simulink model "sim_2"  (R2013b)
settings: Solver=ode3  StartTime=0.0  StopTime=2  MaxStep=0.01  RelTol=1e-3
settings Model: Creator=Ali  LastModifiedBy=Ali

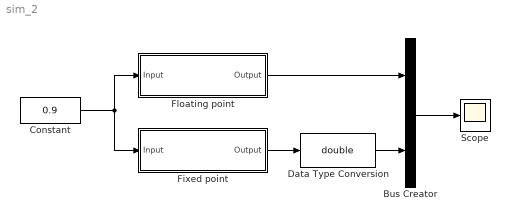
== system sim_2 ==
  Bus Creator : BusCreator  Inputs=2
  Constant : Constant  Value=0.9  SampleTime=Inf
  Data Type Conversion : DataTypeConversion  OutDataTypeStr=double
  Fixed point : Subsystem  Tag=FilterWizardSubSystem
      settings: ErrorFcn=dspFilterRealizedInBasicElemsAlgLoopErrFcnCallback
  Floating point : Subsystem  Tag=FilterWizardSubSystem
      settings: ErrorFcn=dspFilterRealizedInBasicElemsAlgLoopErrFcnCallback
  Scope : Scope
  wires:
  Constant/1 -> Floating point/1(Input), Fixed point/1(Input)
  Floating point/1(Output) -> Bus Creator/1
  Fixed point/1(Output) -> Data Type Conversion/1
  Bus Creator/1 -> Scope/1
  Data Type Conversion/1 -> Bus Creator/2

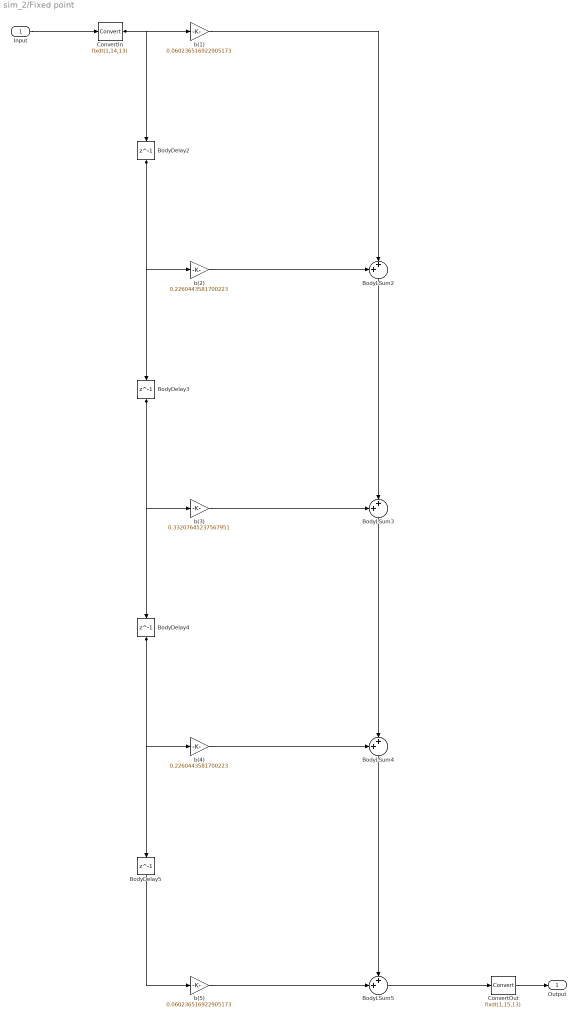
== system sim_2/Fixed point ==
  Input : Inport
  BodyDelay{2..5} (4 alike) : Delay  DelayLength=1  InitialCondition=0  InputProcessing=Columns as channels (frame based)
  BodyLSum{2..5} (4 alike) : Sum  Inputs=++|  AccumDataTypeStr=fixdt(1,22,21)  OutDataTypeStr=fixdt(1,22,21)  RndMeth=Convergent
  ConvertIn : DataTypeConversion  OutDataTypeStr=fixdt(1,14,13)  RndMeth=Nearest  SaturateOnIntegerOverflow=on
  ConvertOut : DataTypeConversion  OutDataTypeStr=fixdt(1,15,13)  RndMeth=Convergent
  b(1) : Gain  Gain=0.060236516922905173  ParamDataTypeStr=fixdt(1,9,8)  OutDataTypeStr=fixdt(1,21,21)  RndMeth=Convergent
  b(2) : Gain  Gain=0.2260443581700223  ParamDataTypeStr=fixdt(1,9,8)  OutDataTypeStr=fixdt(1,21,21)  RndMeth=Convergent
  b(3) : Gain  Gain=0.33207645237567951  ParamDataTypeStr=fixdt(1,9,8)  OutDataTypeStr=fixdt(1,21,21)  RndMeth=Convergent
  b(4) : Gain  Gain=0.2260443581700223  ParamDataTypeStr=fixdt(1,9,8)  OutDataTypeStr=fixdt(1,21,21)  RndMeth=Convergent
  b(5) : Gain  Gain=0.060236516922905173  ParamDataTypeStr=fixdt(1,9,8)  OutDataTypeStr=fixdt(1,21,21)  RndMeth=Convergent
  Output : Outport
  wires:
  Input/1 -> ConvertIn/1
  b(1)/1 -> BodyLSum2/2
  ConvertIn/1 -> b(1)/1, BodyDelay2/1
  BodyDelay2/1 -> b(2)/1, BodyDelay3/1
  b(2)/1 -> BodyLSum2/1
  BodyLSum2/1 -> BodyLSum3/2
  BodyDelay3/1 -> b(3)/1, BodyDelay4/1
  b(3)/1 -> BodyLSum3/1
  BodyLSum3/1 -> BodyLSum4/2
  BodyDelay4/1 -> b(4)/1, BodyDelay5/1
  b(4)/1 -> BodyLSum4/1
  BodyLSum4/1 -> BodyLSum5/1
  BodyDelay5/1 -> b(5)/1
  b(5)/1 -> BodyLSum5/2
  BodyLSum5/1 -> ConvertOut/1
  ConvertOut/1 -> Output/1

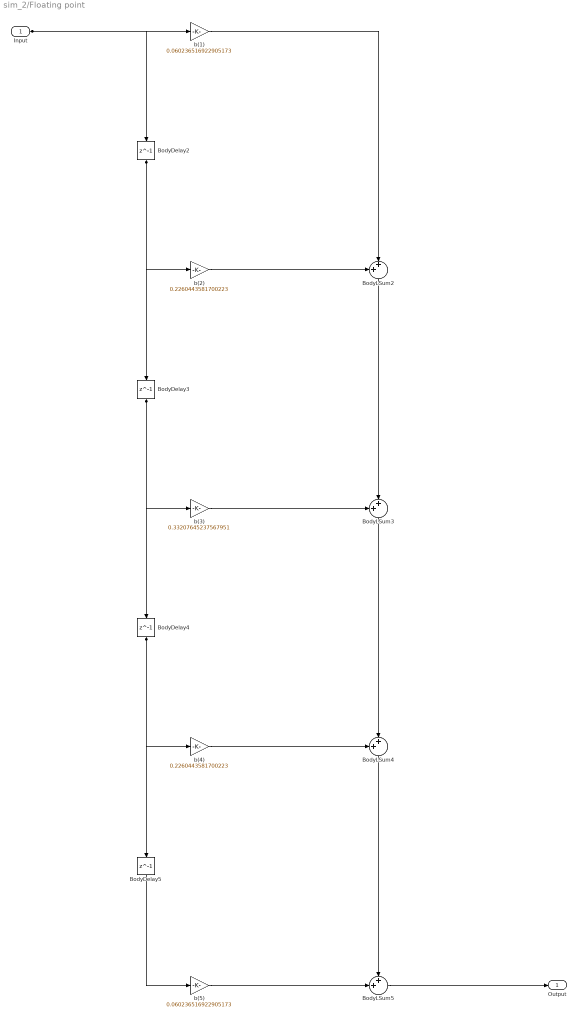
== system sim_2/Floating point ==
  Input : Inport
  BodyDelay{2..5} (4 alike) : Delay  DelayLength=1  InitialCondition=0  InputProcessing=Columns as channels (frame based)
  BodyLSum{2..5} (4 alike) : Sum  Inputs=++|  RndMeth=Nearest  SaturateOnIntegerOverflow=on  OutDataTypeStr=Inherit: Same as first input
  b(1) : Gain  Gain=0.060236516922905173  ParamDataTypeStr=double  RndMeth=Nearest  SaturateOnIntegerOverflow=on  OutDataTypeStr=Inherit: Same as input
  b(2) : Gain  Gain=0.2260443581700223  ParamDataTypeStr=double  RndMeth=Nearest  SaturateOnIntegerOverflow=on  OutDataTypeStr=Inherit: Same as input
  b(3) : Gain  Gain=0.33207645237567951  ParamDataTypeStr=double  RndMeth=Nearest  SaturateOnIntegerOverflow=on  OutDataTypeStr=Inherit: Same as input
  b(4) : Gain  Gain=0.2260443581700223  ParamDataTypeStr=double  RndMeth=Nearest  SaturateOnIntegerOverflow=on  OutDataTypeStr=Inherit: Same as input
  b(5) : Gain  Gain=0.060236516922905173  ParamDataTypeStr=double  RndMeth=Nearest  SaturateOnIntegerOverflow=on  OutDataTypeStr=Inherit: Same as input
  Output : Outport
  wires:
  Input/1 -> b(1)/1, BodyDelay2/1
  b(1)/1 -> BodyLSum2/2
  BodyDelay2/1 -> b(2)/1, BodyDelay3/1
  b(2)/1 -> BodyLSum2/1
  BodyLSum2/1 -> BodyLSum3/2
  BodyDelay3/1 -> b(3)/1, BodyDelay4/1
  b(3)/1 -> BodyLSum3/1
  BodyLSum3/1 -> BodyLSum4/2
  BodyDelay4/1 -> b(4)/1, BodyDelay5/1
  b(4)/1 -> BodyLSum4/1
  BodyLSum4/1 -> BodyLSum5/1
  BodyDelay5/1 -> b(5)/1
  b(5)/1 -> BodyLSum5/2
  BodyLSum5/1 -> Output/1
